simulink model "testNoCollision"  (R2018a)
settings: Solver=VariableStepAuto  StartTime=0.0  StopTime=inf  RelTol=1e-3
InitFcn:
  | run('initArena.m')
undefined symbols (not defined in the file): allObstacles, wall
settings Model: Creator=alex  LastModifiedBy=alex

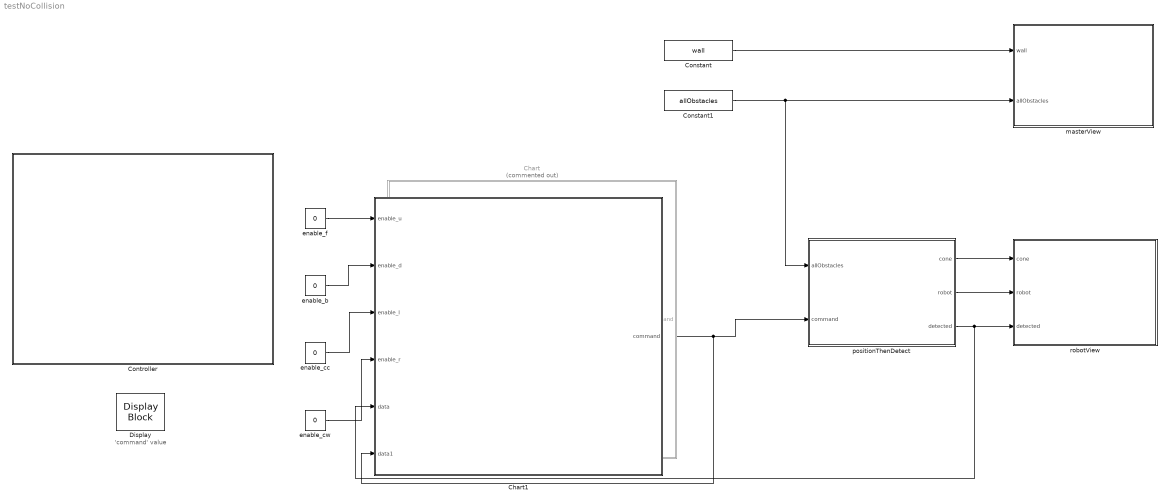
== system testNoCollision ==
  note: 'command' value
  Chart : Stateflow chart  Commented=on  TreatAsAtomicUnit=on
  Chart1 : Stateflow chart  TreatAsAtomicUnit=on
  Constant : Constant  Value=wall
  Constant1 : Constant  Value=allObstacles
  Controller : Subsystem
  Display : DisplayBlock  WebBlockId=14  LabelPosition=Hide
  "enable_b " : Constant  Value=0
  "enable_cc " : Constant  Value=0
  "enable_cw " : Constant  Value=0
  "enable_f " : Constant  Value=0
  masterView : MATLAB Function  TreatAsAtomicUnit=on
  positionThenDetect : MATLAB Function  TreatAsAtomicUnit=on
  robotView : MATLAB Function  TreatAsAtomicUnit=on
  wires:
  "enable_f "/1 -> Chart1/1(enable_u)
  "enable_b "/1 -> Chart1/2(enable_d)
  "enable_cc "/1 -> Chart1/3(enable_l)
  "enable_cw "/1 -> Chart1/4(enable_r)
  Constant/1 -> masterView/1(wall)
  Constant1/1 -> masterView/2(allObstacles), positionThenDetect/1(allObstacles)
  positionThenDetect/1(cone) -> robotView/1(cone)
  positionThenDetect/2(robot) -> robotView/2(robot)
  positionThenDetect/3(detected) -> Chart1/5(data), robotView/3(detected)
  Chart1/1(command) -> Chart1/6(data1), positionThenDetect/2(command)

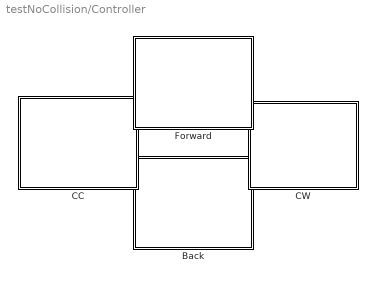
== system testNoCollision/Controller ==
  Back : Subsystem  DialogController=hmiCreateDDGDialog  IsWebBlock=on  mask(MWDashboardBlock){webBlockId=1a5e94ef-030e-49cd-b944-b929b04abc70, webBlockType=pushbutton, ShowInLibBrwoser=on, ShowInitialText=on, HMISrcModelName=noCollision}
      mask prompts: webBlockId "WebBlock Id"; webBlockType "WebBlock Type"; HMISrcModelName "Source Model"
      mask help: SimulinkHMI:dialogs:PushButtonDialogDesc
      mask Help: helpview([docroot '/mapfiles/simulink.map'], 'hmi_push_button')
      mask Display:
      | model = bdroot(gcb);
      | if strcmp(get_param(model,'BlockDiagramType'), 'library')
      |     image([(matlabroot) '/toolbox/simulink/hmi/icons/PushButton.png']);
      | end
  "CC " : Subsystem  DialogController=hmiCreateDDGDialog  IsWebBlock=on  mask(MWDashboardBlock){webBlockId=f6d6ee6b-2047-45ee-ab2e-570b521bf019, webBlockType=pushbutton, ShowInLibBrwoser=on, ShowInitialText=on, HMISrcModelName=noCollision}
      mask prompts: webBlockId "WebBlock Id"; webBlockType "WebBlock Type"; HMISrcModelName "Source Model"
      mask help: SimulinkHMI:dialogs:PushButtonDialogDesc
      mask Help: helpview([docroot '/mapfiles/simulink.map'], 'hmi_push_button')
      mask Display:
      | model = bdroot(gcb);
      | if strcmp(get_param(model,'BlockDiagramType'), 'library')
      |     image([(matlabroot) '/toolbox/simulink/hmi/icons/PushButton.png']);
      | end
  "CW " : Subsystem  DialogController=hmiCreateDDGDialog  IsWebBlock=on  mask(MWDashboardBlock){webBlockId=5b3cd59d-fae2-469c-adcb-5a1af564bf62, webBlockType=pushbutton, ShowInLibBrwoser=on, ShowInitialText=on, HMISrcModelName=noCollision}
      mask prompts: webBlockId "WebBlock Id"; webBlockType "WebBlock Type"; HMISrcModelName "Source Model"
      mask help: SimulinkHMI:dialogs:PushButtonDialogDesc
      mask Help: helpview([docroot '/mapfiles/simulink.map'], 'hmi_push_button')
      mask Display:
      | model = bdroot(gcb);
      | if strcmp(get_param(model,'BlockDiagramType'), 'library')
      |     image([(matlabroot) '/toolbox/simulink/hmi/icons/PushButton.png']);
      | end
  Forward : Subsystem  DialogController=hmiCreateDDGDialog  IsWebBlock=on  mask(MWDashboardBlock){webBlockId=418d2ee9-92ed-471b-995b-1589f387356b, webBlockType=pushbutton, ShowInLibBrwoser=on, ShowInitialText=on, HMISrcModelName=noCollision}
      mask prompts: webBlockId "WebBlock Id"; webBlockType "WebBlock Type"; HMISrcModelName "Source Model"
      mask help: SimulinkHMI:dialogs:PushButtonDialogDesc
      mask Help: helpview([docroot '/mapfiles/simulink.map'], 'hmi_push_button')
      mask Display:
      | model = bdroot(gcb);
      | if strcmp(get_param(model,'BlockDiagramType'), 'library')
      |     image([(matlabroot) '/toolbox/simulink/hmi/icons/PushButton.png']);
      | end

== system testNoCollision/Controller/Back ==

== system testNoCollision/Controller/CC  ==

== system testNoCollision/Controller/CW  ==

== system testNoCollision/Controller/Forward ==

== stateflow chart testNoCollision/Chart1 ==
  state up3
    entry: command = 1
  state down3
    entry: command = 2
  state up2
    entry: command=1
  state left2
    entry: command=3
  state right2
    entry: command=4
  state left3
    entry: command = 3
  state up4
    entry: command = 1
  state down4
    entry: command = 2
  state right4
    entry: command = 4
  state detected_down
    entry: command = 0
  state detected_right
    entry: command = 0
  state detected_left
    entry: command = 0
  state no_input
    entry: command = 0
  state detected_up
    entry: command = 0
  state up
    entry: command = 1
  state down
    entry: command = 2
  state left
    entry: command = 3
  state right
    entry: command = 4
  state down1
    entry:command = 2
  state left1
    entry: command = 3
  state right_1
    entry: command = 4
  detected_down -> up2 [order 2] : [enable_u==1]
  up2 -> detected_down : [enable_u==0]
  detected_down -> left2 [order 4] : [enable_l==1]
  left2 -> detected_down : [enable_l==0]
  right2 -> detected_down : [enable_r==0]
  detected_down -> right2 [order 3] : [enable_r==1]
  detected_right -> up3 [order 3] : [enable_u == 1]
  up3 -> detected_right : [enable_u == 0]
  detected_right -> down3 [order 4] : [enable_d == 1]
  down3 -> detected_right : [enable_d == 0]
  detected_right -> left3 [order 2] : [enable_l == 0]
  left3 -> detected_right : [enable_l == 1]
  detected_left -> up4 [order 3] : [enable_u == 1]
  up4 -> detected_left : [enable_u == 0]
  detected_left -> down4 [order 4] : [enable_d == 1]
  down4 -> detected_left : [enable_d == 0]
  detected_left -> right4 [order 1] : [enable_l == 0]
  detected_up -> no_input [order 3] : [data == 0]
  right4 -> detected_left : [enable_l == 1]
  detected_right -> no_input [order 1] : [data == 0]
  no_input -> detected_right [order 11] : [data == 1]
  no_input -> detected_right [order 12] : [data1 == 4]
  detected_down -> no_input [order 1] : [data == 0]
  no_input -> detected_down [order 9] : [data == 1]
  no_input -> detected_down [order 10] : [data1 == 2]
  (default) -> no_input
  no_input -> detected_up [order 7] : [data==1]
  detected_left -> no_input [order 2] : [data == 0]
  no_input -> detected_left [order 2] : [data == 1]
  no_input -> detected_left [order 3] : [data1 == 3]
  no_input -> detected_up [order 8] : [data1 == 1]
  no_input -> up [order 6] : [enable_u == 1]
  up -> no_input : [enable_u == 0]
  no_input -> down [order 5] : [enable_d ==1]
  down -> no_input : [enable_d == 0]
  no_input -> left [order 4] : [enable_l == 1]
  left -> no_input : [enable_l == 0]
  no_input -> right [order 1] : [enable_r == 1]
  right -> no_input : [enable_r == 0]
  down1 -> detected_up : [enable_d == 0]
  right_1 -> detected_up [order 2] : [enable_r == 0]
  right_1 -> detected_up [order 1] : [enable_r == 1]
  detected_up -> down1 [order 1] : [enable_d ==1]
  detected_up -> left1 [order 2] : [enable_l == 1]
  left1 -> detected_up : [enable_l == 0]
  data: enable_u input; enable_d input; enable_l input; enable_r input; command output; data input; data1 input

== matlab function testNoCollision/positionThenDetect ==
  data: allObstacles input; cone output; command input; robot output; detected output
function [cone, robot, detected] = positionThenDetect(allObstacles, command)
    persistent xpos ypos
    if isempty(xpos)
        xpos = 2000;
        ypos = 2000;
    end
    
    % Base vision cone 
    line1 = [0,150,0; 300,450,0;];
    line2 = [0,150,0; -300,450,0;];
    line3 = [-300,450,0; 300,450,0;];
    base_cone = vertcat(line1, line2, line3);
    
    % Base robot 
    xbase_robot = [0, -100, -100, +100, 100, 0];
    ybase_robot = [150, 50, -150, -150, 50, 150];
    
    % Translate base cone and base robot based on x and y position
    if command == 1
        ypos = ypos + 50;
    elseif command == 2
        ypos = ypos - 50;
    elseif command == 3
        xpos = xpos - 50;
    elseif command == 4
        xpos = xpos + 50;
    end

    cone = base_cone;
    cone(:,1) = base_cone(:,1) + xpos;
    cone(:,2) = base_cone(:,2) + ypos;
    cone(:,3) = base_cone(:,3);

    xrobot = xbase_robot + xpos;
    yrobot = ybase_robot + ypos;
    robot = fliplr(rot90(vertcat(xrobot,yrobot),3));

    % Check if obstacle is in vision cone 
    detected = detectObject(allObstacles, cone); 
end

== stateflow chart testNoCollision/Chart ==
  state no_input
    entry: command = 0
  state forward
    entry: command = 1
  state back
    entry: command = 2
  state counter_clockwise
    entry: command = 3
  state clockwise
    entry: command = 4
  (default) -> no_input
  no_input -> forward [order 4] : [enable_f == 1]
  forward -> no_input : [enable_f == 0]
  no_input -> back [order 3] : [enable_b ==1]
  back -> no_input : [enable_b== 0]
  no_input -> counter_clockwise [order 2] : [enable_cc == 1]
  counter_clockwise -> no_input : [enable_cc == 0]
  no_input -> clockwise [order 1] : [enable_cw == 1]
  clockwise -> no_input : [enable_cw == 0]
  data: enable_f input; enable_b input; enable_cc input; enable_cw input; command output

== matlab function testNoCollision/masterView ==
  data: wall input; allObstacles input
function masterView(wall, allObstacles)
    % Visualize data 
    % hold on
    grid on
    grid minor
    xlim([-800 6600])
    ylim([-700 4400])
    plot(wall(:,1), wall(:,2), 'ks-');
    hold on 
    plot(allObstacles(:,1), allObstacles(:,2), 'bs');
end

== matlab function testNoCollision/robotView ==
  data: cone input; robot input; detected input
function robotView(cone, robot, detected) 
     if detected
        coneColor = 'r.-';
    else
        coneColor = 'k.-';
    end
    coneFig = plot(cone(:,1), cone(:,2), coneColor); 
    botFig = plot(robot(:,1), robot(:,2), 'k.-');
    set([coneFig botFig],'LineWidth', 5)
    hold off
end
